simulink model "LoadSaveCycleControl_test"  (Simulink 6.2)
settings: Solver=FixedStepDiscrete  StartTime=0.0  StopTime=3  FixedStep=1  RelTol=1e-3
values from neighbouring files (symbols this model uses):
  parameters = getappdata(handles.parameter_GUI, 'Parameter_Data')    [LoadSaveCycleControl_GUI.m]
libraries: LoadSaveCycleControl_lib x1
settings Model: LastModifiedBy=bsaunder
settings DebuggingCC: SolverPrmCheckMsg=warning

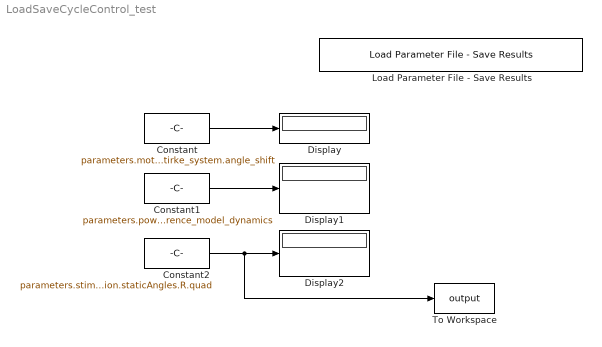
== system LoadSaveCycleControl_test ==
  Constant : Constant  Value=parameters.motor_tirke_system.angle_shift
  Constant1 : Constant  Value=parameters.power_control_design.reference_model_dynamics
  Constant2 : Constant  Value=parameters.stimulation.staticAngles.R.quad
  Display : Display
  Display1 : Display
  Display2 : Display
  Load Parameter File - Save Results : LoadSaveCycleControl_lib/Load Parameter File - Save Results
  To Workspace : ToWorkspace  VariableName=output  SampleTime=-1  SaveFormat=Array
  wires:
  Constant/1 -> Display/1
  Constant1/1 -> Display1/1
  Constant2/1 -> Display2/1, To Workspace/1
